simulink model "block_yawrate"  (R2019b)
settings: Solver=VariableStepAuto  StartTime=0.0  StopTime=10.0  RelTol=1e-3
values from neighbouring files (symbols this model uses):
  Iz = 1500    [block_params.mat]    (also in coefficien.m; params.mat)
  Kf = 50000    [block_params.mat]    (also in coefficien.m; params.mat)
  Kr = 50000    [block_params.mat]    (also in coefficien.m; params.mat)
  lf = 1.2    [block_params.mat]    (also in coefficien.m; params.mat)
  lr = 1.4    [block_params.mat]    (also in coefficien.m; params.mat)
  m = 1200    [block_params.mat]    (also in coefficien.m; params.mat; params_stock.m = 10)
  V = [8.33333333333 16.6666666667 25 33.3333333333 41.6666666667 50]    [block_params.mat]    (also in coefficien.m = [30:30:180]/3.6; coefficien_lateral_accelration.m = V*(1000/(60*60)); coefficien_sideslip_angre.m = V*(1000/(60*60)); coefficien_turning_trajectory.m = V*(1000/(60*60)))
settings Model: Creator=Peanatsu  LastModifiedBy=Peanatsu

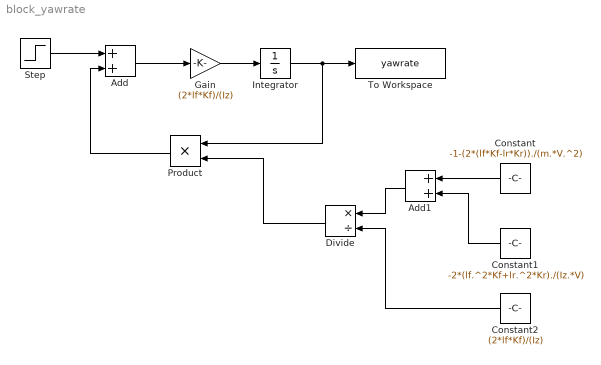
== system block_yawrate ==
  Add : Sum
  Add1 : Sum
  Constant : Constant  Value=-1-(2*(lf*Kf-lr*Kr))./(m.*V.^2)
  Constant1 : Constant  Value=-2*(lf.^2*Kf+lr.^2*Kr)./(Iz.*V)
  Constant2 : Constant  Value=(2*lf*Kf)/(Iz)
  Divide : Product  Inputs=*/
  Gain : Gain  Gain=(2*lf*Kf)/(Iz)
  Integrator : Integrator
  Product : Product
  Step : Step  Time=0  SampleTime=0
  To Workspace : ToWorkspace  VariableName=yawrate  SaveFormat=Timeseries  SampleTime=-1
  wires:
  Step/1 -> Add/1
  Add/1 -> Gain/1
  Gain/1 -> Integrator/1
  Integrator/1 -> Product/1, To Workspace/1
  Product/1 -> Add/2
  Constant/1 -> Add1/1
  Constant1/1 -> Add1/2
  Add1/1 -> Divide/1
  Constant2/1 -> Divide/2
  Divide/1 -> Product/2
